simulink model "test_XY2WGS_sensor"  (R2025a)
settings: Solver=VariableStepAuto  StartTime=0.0  StopTime=10.0  RelTol=1e-3  AbsTol=1e-3
PostLoadFcn:
  | Coords = Coords_WGSTest;
libraries: nesl_utility x1
Description:
  | Copyright 2024-2025 The MathWorks, Inc.
settings Model: Creator=smiller  LastModifiedBy=smiller
settings SolverCC: AutoScaleAbsTol=off  AlgebraicLoopSolver=TrustRegion  MaxZcPerStep=1.0
settings OptimizationCC: ReuseModelBlockBuffer=off
settings DebuggingCC: UnconnectedInputMsg=warning  UnconnectedOutputMsg=warning  UnconnectedLineMsg=warning  SymbolicDimsDataTypeCodeGenerationDiagnostic=none
settings ModelReferenceCC: EnableRefExpFcnMdlSchedulingChecks=on
settings SFSimCC: CustomCodeUndefinedFunction=UseInterfaceOnly
settings RTWCC: GPUComputeCapability=3.5  DLArmComputeVersion=19.05
settings SimscapeCC: SimscapeLogType=all  SimscapeLogSimulationStatistics=on  SimscapeLogDataHistory=10000.0

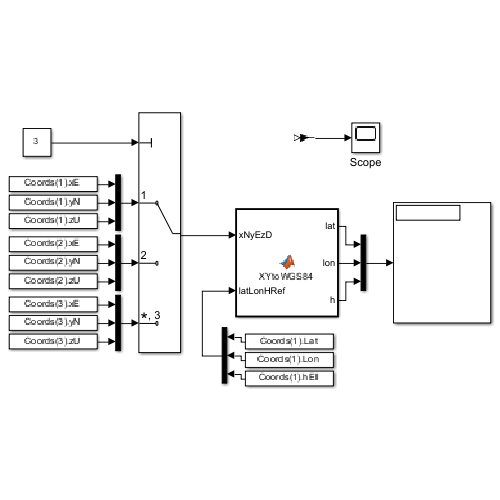
[thumbnail: Simulink's stored preview of the top-level diagram]
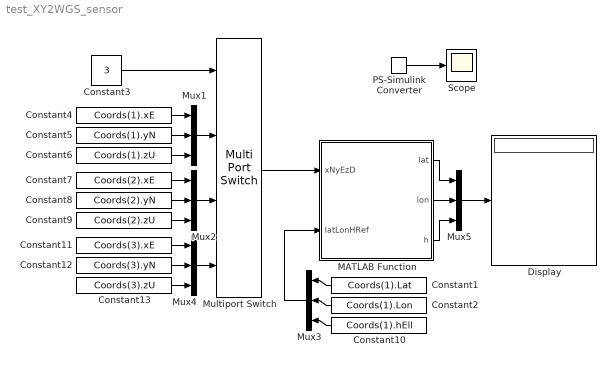
== system test_XY2WGS_sensor ==
  Constant1 : Constant  Value=Coords(1).Lat
  Constant10 : Constant  Value=Coords(1).hEll
  Constant11 : Constant  Value=Coords(3).xE
  Constant12 : Constant  Value=Coords(3).yN
  Constant13 : Constant  Value=Coords(3).zU
  Constant2 : Constant  Value=Coords(1).Lon
  Constant3 : Constant  Value=3
  Constant4 : Constant  Value=Coords(1).xE
  Constant5 : Constant  Value=Coords(1).yN
  Constant6 : Constant  Value=Coords(1).zU
  Constant7 : Constant  Value=Coords(2).xE
  Constant8 : Constant  Value=Coords(2).yN
  Constant9 : Constant  Value=Coords(2).zU
  Display : Display
  MATLAB Function : MATLAB Function  TreatAsAtomicUnit=on
  Multiport Switch : MultiPortSwitch  SaturateOnIntegerOverflow=off  InputSameDT=off
  Mux{1..5} (5 alike) : Mux  Inputs=3
  PS-Simulink Converter : nesl_utility/PS-Simulink Converter  PhysicalDomain=network_engine_domain  SubClassName=ps_output  LeftPortType=input  RightPortType=output  PseudoPeriodic=off  Frequencies=[]  VectorFormat=inherit  Unit=inherit  AffineConversion=off
  Scope : Scope
  wires:
  PS-Simulink Converter/1 -> Scope/1
  Mux3/1 -> MATLAB Function/2(latLonHRef)
  Multiport Switch/1 -> MATLAB Function/1(xNyEzD)
  Mux1/1 -> Multiport Switch/2
  Constant6/1 -> Mux1/3
  Constant5/1 -> Mux1/2
  Constant4/1 -> Mux1/1
  Constant7/1 -> Mux2/1
  Constant8/1 -> Mux2/2
  Constant9/1 -> Mux2/3
  Mux2/1 -> Multiport Switch/3
  Constant1/1 -> Mux3/1
  Constant2/1 -> Mux3/2
  Constant10/1 -> Mux3/3
  Constant13/1 -> Mux4/3
  Constant12/1 -> Mux4/2
  Constant11/1 -> Mux4/1
  Mux4/1 -> Multiport Switch/4
  Constant3/1 -> Multiport Switch/1
  MATLAB Function/1(lat) -> Mux5/1
  MATLAB Function/3(h) -> Mux5/3
  MATLAB Function/2(lon) -> Mux5/2
  Mux5/1 -> Display/1

== matlab function test_XY2WGS_sensor/MATLAB Function ==
  data: xNyEzD input; lat output; latLonHRef input; lon output; h output
function [lat, lon, h] = XYtoWGS84(xNyEzD,latLonHRef)

[lat, lon, h] = ned2geodetic(...
    xNyEzD(1),xNyEzD(2),xNyEzD(3),...
    latLonHRef(1),latLonHRef(2),latLonHRef(3),...
    wgs84Ellipsoid);
